simulink library "Controls_Components_lib"  (R2023b)
settings: Solver=VariableStepAuto  StartTime=0.0  StopTime=10.0  RelTol=1e-3
libraries: simulink x15, $bdroot x4, simulink_extras x3, simulink_need_slupdate x2, embmathops x1
settings Model: Creator=FIRSTMentor  LastModifiedBy=FIRSTMentor

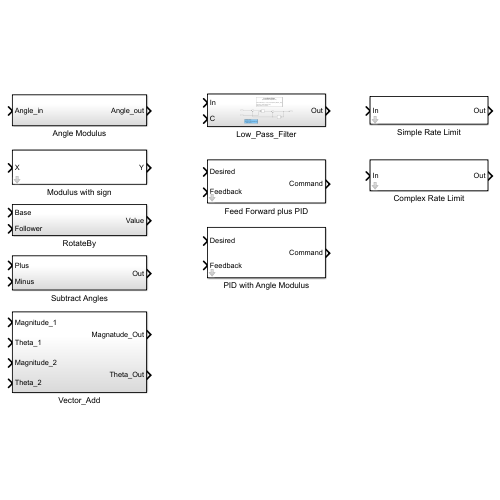
[thumbnail: Simulink's stored preview of the top-level diagram]
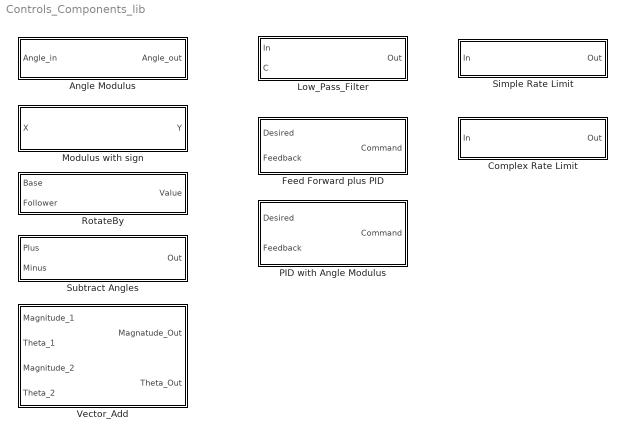
== system Controls_Components_lib ==
  Angle Modulus : Subsystem
  Complex Rate Limit : Subsystem  mask{Rate_Limit_Inc=1/0.75*0.02, Rate_Limit_Dec=-1/0.25*0.02, Approaching_Zero_Error_Threshold=0.2, Approaching_Zero_Final_Scale_Factor=0.01, Approaching_NonZero_Error_Threshold=0.2, Approaching_NonZero_Final_Scale_Factor=0.1}
  Feed Forward plus PID : Subsystem  mask{Gain_FF=1, Gain_P=1, Gain_I=1, Gain_D=1, FilterCoeff_D=0.1, Limit_I_Upper=0.1, Limit_I_Lower=-0.1, Limit_D_Upper=0.1, Limit_D_Lower=-0.1, Limit_T_Upper=1, Limit_T_Lower=-1}
      mask prompts: Gain_FF "Feed Forward Gain"; Gain_P "Proportional Gain"; Gain_I "Integral Gain"; Gain_D "Derivative Gain"; FilterCoeff_D "Derivative Filter Coefficient"; Limit_I_Upper "Integral Upper Limit"; Limit_I_Lower "Integral Lower Limit"; Limit_D_Upper "Derivative Upper Limit"; Limit_D_Lower "Derivative Lower Limit"; Limit_T_Upper "Total Command Upper Limit"; Limit_T_Lower "Total Command Lower Limit"
  Low_Pass_Filter : Subsystem
  Modulus with sign : Subsystem  mask{Number=1}
      mask prompts: Number "Enter modulus number"
  PID with Angle Modulus : Subsystem  mask{Gain_P=1, Gain_I=1, Gain_D=1, FilterCoeff_D=0.1, Limit_I_Upper=0.1, Limit_I_Lower=-0.1, Limit_D_Upper=0.1, Limit_D_Lower=-0.1, Limit_T_Upper=1, Limit_T_Lower=-1}
      mask prompts: Gain_P "Proportional Gain"; Gain_I "Integral Gain"; Gain_D "Derivative Gain"; FilterCoeff_D "Derivative Filter Coefficient"; Limit_I_Upper "Integral Upper Limit"; Limit_I_Lower "Integral Lower Limit"; Limit_D_Upper "Derivative Upper Limit"; Limit_D_Lower "Derivative Lower Limit"; Limit_T_Upper "Total Command Upper Limit"; Limit_T_Lower "Total Command Lower Limit"
  RotateBy : Subsystem
  Simple Rate Limit : Subsystem  mask{Rate_Limit_Inc=1/0.75*0.02, Rate_Limit_Dec=-1/0.25*0.02}
  Subtract Angles : Subsystem
  Vector_Add : Subsystem

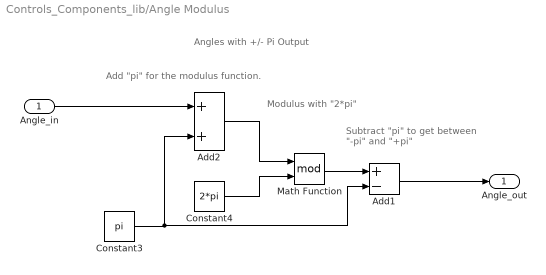
== system Controls_Components_lib/Angle Modulus ==
  note: Angles with +/- Pi Output
  note: Subtract "pi" to get
      | between "-pi" and "+pi"
  note: Modulus with "2*pi"
  note: Add "pi" for the modulus function.
  Angle_in : Inport
  Add1 : Sum  Inputs=+-
  Add2 : Sum
  Constant3 : Constant  Value=pi
  Constant4 : Constant  Value=2*pi
  Math Function : Math  Operator=mod
  Angle_out : Outport
  wires:
  Add1/1 -> Angle_out/1
  Math Function/1 -> Add1/1
  Constant4/1 -> Math Function/2
  Add2/1 -> Math Function/1
  Constant3/1 -> Add2/2, Add1/2
  Angle_in/1 -> Add2/1

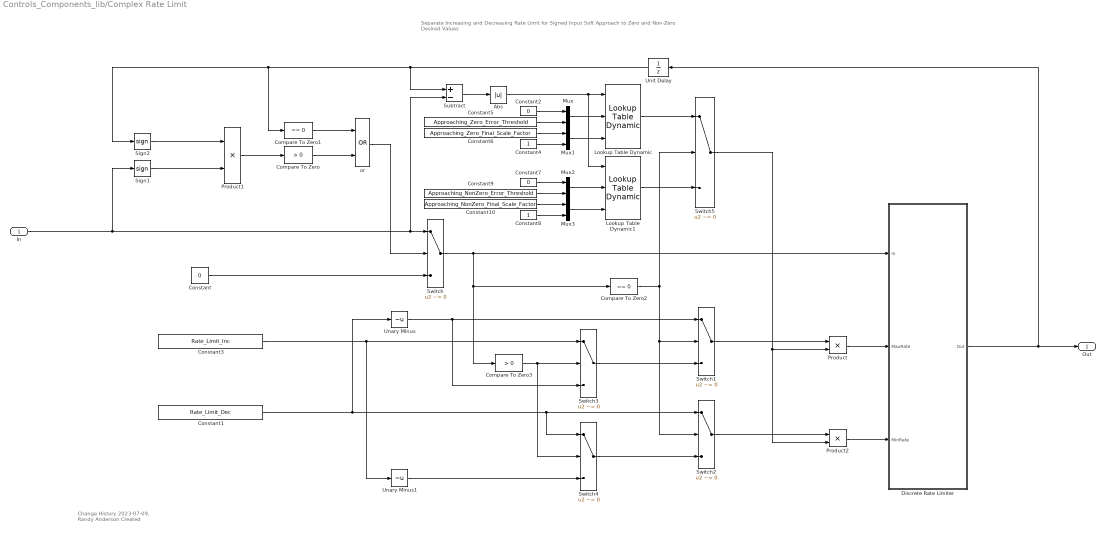
== system Controls_Components_lib/Complex Rate Limit ==
  note: Separate Increasing and Decreasing Rate Limit for Signed Input
      | Soft Approach to Zero and Non-Zero Desired Values
  note: Change History
      | 2023-07-09, Randy Anderson
      |     Created
  In : Inport
  Abs : Abs  SaturateOnIntegerOverflow=off
  Compare To Zero : simulink/Logic and Bit Operations/Compare To Zero  relop=>  OutDataTypeStr=boolean
      settings: AttributesFormatString=%<OutDataTypeStr>
  Compare To Zero1 : simulink/Logic and Bit Operations/Compare To Zero  relop===  OutDataTypeStr=boolean
      settings: AttributesFormatString=%<OutDataTypeStr>
  Compare To Zero2 : simulink/Logic and Bit Operations/Compare To Zero  relop===  OutDataTypeStr=boolean
      settings: AttributesFormatString=%<OutDataTypeStr>
  Compare To Zero3 : simulink/Logic and Bit Operations/Compare To Zero  relop=>  OutDataTypeStr=boolean
      settings: AttributesFormatString=%<OutDataTypeStr>
  Constant : Constant  Value=0  OutDataTypeStr=Inherit: Inherit via back propagation
      settings: AttributesFormatString=%<OutDataTypeStr>
  Constant1 : Constant  Value=Rate_Limit_Dec
      settings: AttributesFormatString=%<OutDataTypeStr>
  Constant10 : Constant  Value=Approaching_NonZero_Final_Scale_Factor
  Constant2 : Constant  Value=0
  Constant3 : Constant  Value=Rate_Limit_Inc
      settings: AttributesFormatString=%<OutDataTypeStr>
  Constant4 : Constant
  Constant5 : Constant  Value=Approaching_Zero_Error_Threshold
  Constant6 : Constant  Value=Approaching_Zero_Final_Scale_Factor
  Constant7 : Constant  Value=0
  Constant8 : Constant
  Constant9 : Constant  Value=Approaching_NonZero_Error_Threshold
  Discrete Rate Limiter : Subsystem
  Lookup Table Dynamic : simulink/Lookup Tables/Lookup Table Dynamic  LookUpMeth=Interpolation-Use End Values  OutDataType=fixdt('double')  OutScaling=[]  OutputDataTypeScalingMode=Specify via dialog  OutDataTypeStr=double  DoSatur=off
  Lookup Table Dynamic1 : simulink/Lookup Tables/Lookup Table Dynamic  LookUpMeth=Interpolation-Use End Values  OutDataType=fixdt('double')  OutScaling=[]  OutputDataTypeScalingMode=Specify via dialog  OutDataTypeStr=double  DoSatur=off
  Mux{,1..3} (4 alike) : Mux  Inputs=2
  Product : Product
  Product1 : Product  OutDataTypeStr=int8  RndMeth=Simplest
      settings: AttributesFormatString=Input Same DT: %<InputSameDT>\n%<OutDataTypeStr>\nSaturate: %<SaturateOnIntegerOverflow>
  Product2 : Product
  Sign1 : Signum
  Sign2 : Signum
  Subtract : Sum  Inputs=+-
  Switch{,1..4} (5 alike) : Switch  Criteria=u2 ~= 0  SaturateOnIntegerOverflow=off
      settings: AttributesFormatString=|
      | %<Criteria>
      | Input Same DT: %<InputSameDT>
      | %<OutDataTypeStr>
  Switch5 : Switch  Criteria=u2 ~= 0  SaturateOnIntegerOverflow=off  InputSameDT=off
  Unary Minus : UnaryMinus
  Unary Minus1 : UnaryMinus
  Unit Delay : UnitDelay  SampleTime=-1  HasFrameUpgradeWarning=on
      settings: AttributesFormatString=IC: %<InitialCondition>
  or : Logic  Operator=OR  OutDataTypeStr=boolean
      settings: AttributesFormatString=|
      | Input Same DT: %<AllPortsSameDT>
      | %<OutDataTypeStr>
  Out : Outport
  wires:
  Unary Minus1/1 -> Switch4/3
  Constant3/1 -> Switch3/1, Unary Minus1/1
  Unary Minus/1 -> Switch1/1, Switch3/3
  Constant1/1 -> Switch2/1, Switch4/1, Unary Minus/1
  Compare To Zero3/1 -> Switch3/2, Switch4/2
  Switch4/1 -> Switch2/3
  Switch3/1 -> Switch1/3
  Compare To Zero2/1 -> Switch2/2, Switch1/2, Switch5/2
  Compare To Zero1/1 -> or/1
  or/1 -> Switch/2
  Compare To Zero/1 -> or/2
  Discrete Rate Limiter/1(Out) -> Out/1, Unit Delay/1
  Sign1/1 -> Product1/2
  Sign2/1 -> Product1/1
  Unit Delay/1 -> Subtract/1, Compare To Zero1/1, Sign2/1
  Product1/1 -> Compare To Zero/1
  Switch/1 -> Compare To Zero2/1, Compare To Zero3/1, Discrete Rate Limiter/1(In)
  In/1 -> Sign1/1, Subtract/2, Switch/1
  Constant/1 -> Switch/3
  Switch1/1 -> Product/1
  Product/1 -> Discrete Rate Limiter/2(MaxRate)
  Product2/1 -> Discrete Rate Limiter/3(MinRate)
  Switch2/1 -> Product2/1
  Subtract/1 -> Abs/1
  Abs/1 -> Lookup Table Dynamic1/1, Lookup Table Dynamic/1
  Switch5/1 -> Product/2, Product2/2
  Lookup Table Dynamic/1 -> Switch5/1
  Mux/1 -> Lookup Table Dynamic/2
  Mux1/1 -> Lookup Table Dynamic/3
  Constant2/1 -> Mux/1
  Constant4/1 -> Mux1/2
  Constant5/1 -> Mux/2
  Constant6/1 -> Mux1/1
  Constant10/1 -> Mux3/1
  Constant9/1 -> Mux2/2
  Constant8/1 -> Mux3/2
  Constant7/1 -> Mux2/1
  Mux3/1 -> Lookup Table Dynamic1/3
  Mux2/1 -> Lookup Table Dynamic1/2
  Lookup Table Dynamic1/1 -> Switch5/3

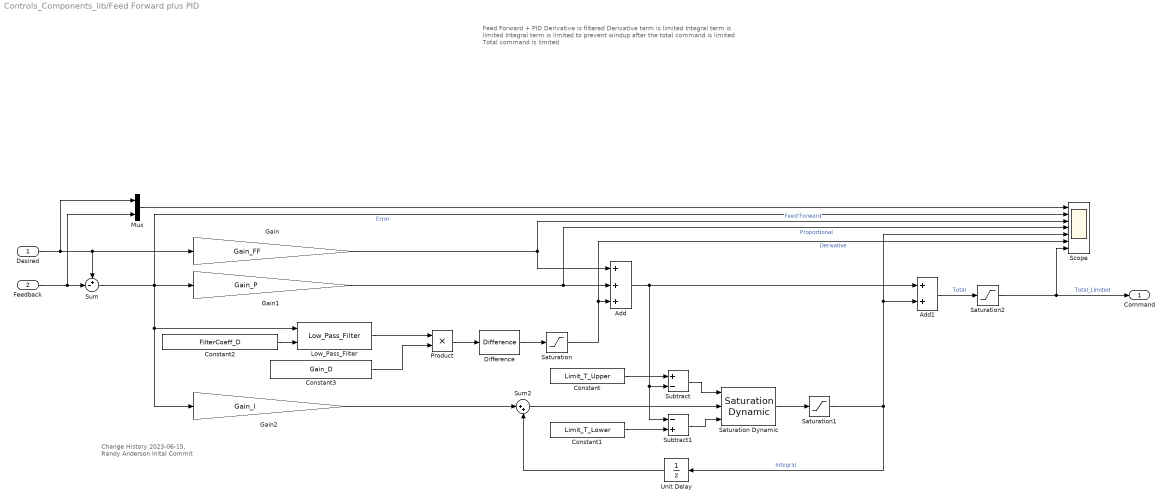
== system Controls_Components_lib/Feed Forward plus PID ==
  note: Feed Forward + PID
      |
      | Derivative is filtered
      | Derivative term is limited
      |
      | Integral term is limited
      |
      | Integral term is limited to prevent windup after the total command is limited
      |
      | Total command is limited
  note: Change History
      | 2023-06-15, Randy Anderson
      | Inital Commit
  Desired : Inport
  Feedback : Inport  Port=2
  Add : Sum  Inputs=3
  Add1 : Sum  Inputs=2
  Constant : Constant  Value=Limit_T_Upper
  Constant1 : Constant  Value=Limit_T_Lower
  Constant2 : Constant  Value=FilterCoeff_D
  Constant3 : Constant  Value=Gain_D
  Difference : simulink/Discrete/Difference  ICPrevInput=0.0  OutMin=[]  OutMax=[]  OutDataType=fixdt(1, 16)  OutScaling=2^-10  DoSatur=off
  Gain : Gain  Gain=Gain_FF
  Gain1 : Gain  Gain=Gain_P
  Gain2 : Gain  Gain=Gain_I
  Low_Pass_Filter : $bdroot/Low_Pass_Filter  SystemSampleTime=-1  VariantActivationTime=update diagram  AllowFlexibleInterface=on  Latency=0  AutoFrameSizeCalculation=off
  Mux : Mux  Inputs=2
  Product : Product
  Saturation : Saturate  UpperLimit=Limit_D_Upper  LowerLimit=Limit_D_Lower
  Saturation Dynamic : simulink/Discontinuities/Saturation Dynamic  OutMin=[]  OutMax=[]  OutDataTypeStr=Inherit: Same as second input  OutDataType=fixdt(1, 16)  OutScaling=2^-10  DoSatur=off
  Saturation1 : Saturate  UpperLimit=Limit_I_Upper  LowerLimit=Limit_I_Lower
  Saturation2 : Saturate  UpperLimit=Limit_T_Upper  LowerLimit=Limit_T_Lower
  Scope : Scope  NumInputPorts=7
  Subtract : Sum  Inputs=+-
  Subtract1 : Sum  Inputs=-+
  Sum : Sum  Inputs=+-|
  Sum2 : Sum  Inputs=|++
  Unit Delay : UnitDelay  SampleTime=-1  HasFrameUpgradeWarning=on
  Command : Outport
  wires:
  Sum/1 -> Gain2/1, Low_Pass_Filter/1, Gain1/1, Scope/2  "Error"
  Gain/1 -> Add/1, Scope/3  "Feed Forward"
  Add/1 -> Add1/1, Subtract1/1, Subtract/2
  Subtract1/1 -> Saturation Dynamic/3
  Gain1/1 -> Add/2, Scope/4  "Proportional"
  Gain2/1 -> Sum2/1
  Saturation Dynamic/1 -> Saturation1/1
  Subtract/1 -> Saturation Dynamic/1
  Unit Delay/1 -> Sum2/2
  Constant/1 -> Subtract/1
  Constant1/1 -> Subtract1/2
  Add1/1 -> Saturation2/1  "Total"
  Desired/1 -> Mux/1, Sum/1, Gain/1
  Difference/1 -> Saturation/1
  Saturation/1 -> Scope/6, Add/3  "Derivative"
  Product/1 -> Difference/1
  Low_Pass_Filter/1 -> Product/1
  Constant2/1 -> Low_Pass_Filter/2
  Constant3/1 -> Product/2
  Sum2/1 -> Saturation Dynamic/2
  Feedback/1 -> Mux/2, Sum/2
  Saturation2/1 -> Scope/7, Command/1  "Total_Limited"
  Saturation1/1 -> Unit Delay/1, Scope/5, Add1/2  "Integral"
  Mux/1 -> Scope/1

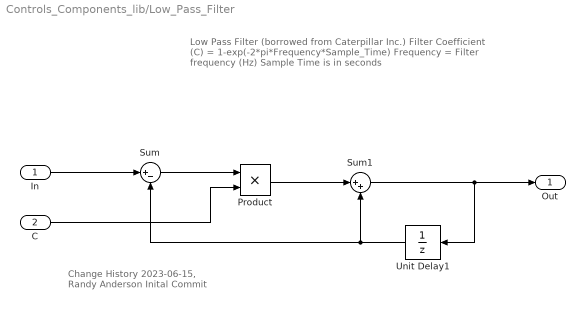
== system Controls_Components_lib/Low_Pass_Filter ==
  note: Low Pass Filter
      | (borrowed from Caterpillar Inc.)
      |
      | Filter Coefficient (C) = 1-exp(-2*pi*Frequency*Sample_Time)
      |
      | Frequency = Filter frequency (Hz)
      | Sample Time is in seconds
  note: Change History
      | 2023-06-15, Randy Anderson
      | Inital Commit
  In : Inport
  C : Inport  Port=2
  Product : Product
  Sum : Sum  Inputs=|+-
  Sum1 : Sum  Inputs=|++
  Unit Delay1 : UnitDelay  SampleTime=-1  HasFrameUpgradeWarning=on
  Out : Outport
  wires:
  In/1 -> Sum/1
  Sum1/1 -> Out/1, Unit Delay1/1
  Product/1 -> Sum1/1
  Unit Delay1/1 -> Sum/2, Sum1/2
  Sum/1 -> Product/1
  C/1 -> Product/2

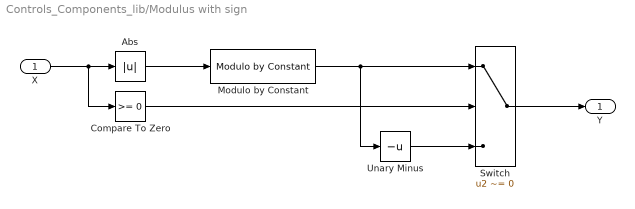
== system Controls_Components_lib/Modulus with sign ==
  X : Inport
  Abs : Abs  SaturateOnIntegerOverflow=off
  Compare To Zero : simulink/Logic and Bit Operations/Compare To Zero  relop=>=  OutDataTypeStr=boolean
  Modulo by Constant : embmathops/Modulo by Constant  Denominator=Number  SimulateUsing=Code generation
      settings: LibrarySourceBlock=embeddedMathLib/Modulo by Constant
  Switch : Switch  Criteria=u2 ~= 0  SaturateOnIntegerOverflow=off  InputSameDT=off
  Unary Minus : UnaryMinus
  Y : Outport
  wires:
  X/1 -> Compare To Zero/1, Abs/1
  Abs/1 -> Modulo by Constant/1
  Switch/1 -> Y/1
  Modulo by Constant/1 -> Unary Minus/1, Switch/1
  Unary Minus/1 -> Switch/3
  Compare To Zero/1 -> Switch/2

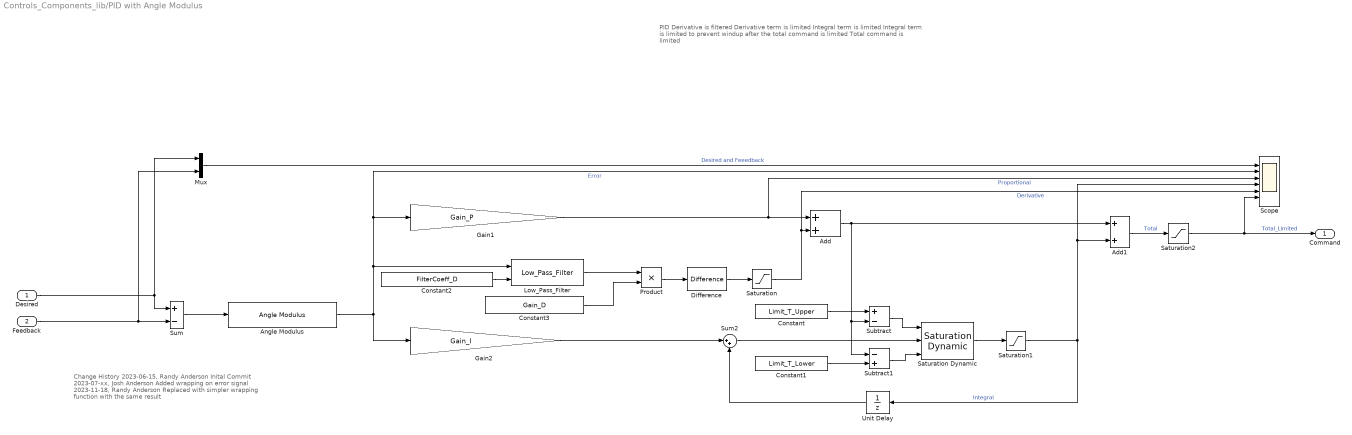
== system Controls_Components_lib/PID with Angle Modulus ==
  note: PID
      |
      | Derivative is filtered
      | Derivative term is limited
      |
      | Integral term is limited
      |
      | Integral term is limited to prevent windup after the total command is limited
      |
      | Total command is limited
  note: Change History
      | 2023-06-15, Randy Anderson
      | Inital Commit
      | 2023-07-xx, Josh Anderson
      | Added wrapping on error signal
      | 2023-11-18, Randy Anderson
      | Replaced with simpler wrapping function with the same result
  Desired : Inport
  Feedback : Inport  Port=2
  Add : Sum  Inputs=2
  Add1 : Sum  Inputs=2
  Angle Modulus : $bdroot/Angle Modulus  SystemSampleTime=-1  VariantActivationTime=update diagram  AllowFlexibleInterface=on  Latency=0  AutoFrameSizeCalculation=off
  Constant : Constant  Value=Limit_T_Upper
  Constant1 : Constant  Value=Limit_T_Lower
  Constant2 : Constant  Value=FilterCoeff_D
  Constant3 : Constant  Value=Gain_D
  Difference : simulink/Discrete/Difference  ICPrevInput=0.0  OutMin=[]  OutMax=[]  OutDataType=fixdt(1, 16)  OutScaling=2^-10  DoSatur=off
  Gain1 : Gain  Gain=Gain_P
  Gain2 : Gain  Gain=Gain_I
  Low_Pass_Filter : $bdroot/Low_Pass_Filter  SystemSampleTime=-1  VariantActivationTime=update diagram  AllowFlexibleInterface=on  Latency=0  AutoFrameSizeCalculation=off
  Mux : Mux  Inputs=2
  Product : Product
  Saturation : Saturate  UpperLimit=Limit_D_Upper  LowerLimit=Limit_D_Lower
  Saturation Dynamic : simulink/Discontinuities/Saturation Dynamic  OutMin=[]  OutMax=[]  OutDataTypeStr=Inherit: Same as second input  OutDataType=fixdt(1, 16)  OutScaling=2^-10  DoSatur=off
  Saturation1 : Saturate  UpperLimit=Limit_I_Upper  LowerLimit=Limit_I_Lower
  Saturation2 : Saturate  UpperLimit=Limit_T_Upper  LowerLimit=Limit_T_Lower
  Scope : Scope  NumInputPorts=6
  Subtract : Sum  Inputs=+-
  Subtract1 : Sum  Inputs=-+
  Sum : Sum  Inputs=+-
  Sum2 : Sum  Inputs=|++
  Unit Delay : UnitDelay  SampleTime=-1  HasFrameUpgradeWarning=on
  Command : Outport
  wires:
  Angle Modulus/1 -> Gain1/1, Scope/2, Low_Pass_Filter/1, Gain2/1  "Error"
  Add/1 -> Subtract1/1, Subtract/2, Add1/1
  Subtract1/1 -> Saturation Dynamic/3
  Gain1/1 -> Scope/3, Add/1  "Proportional"
  Gain2/1 -> Sum2/1
  Saturation Dynamic/1 -> Saturation1/1
  Subtract/1 -> Saturation Dynamic/1
  Unit Delay/1 -> Sum2/2
  Constant/1 -> Subtract/1
  Constant1/1 -> Subtract1/2
  Add1/1 -> Saturation2/1  "Total"
  Desired/1 -> Mux/1, Sum/1
  Difference/1 -> Saturation/1
  Saturation/1 -> Scope/5, Add/2  "Derivative"
  Product/1 -> Difference/1
  Low_Pass_Filter/1 -> Product/1
  Constant2/1 -> Low_Pass_Filter/2
  Constant3/1 -> Product/2
  Sum2/1 -> Saturation Dynamic/2
  Feedback/1 -> Mux/2, Sum/2
  Saturation2/1 -> Scope/6, Command/1  "Total_Limited"
  Saturation1/1 -> Unit Delay/1, Scope/4, Add1/2  "Integral"
  Mux/1 -> Scope/1  "Desired and Feeedback"
  Sum/1 -> Angle Modulus/1

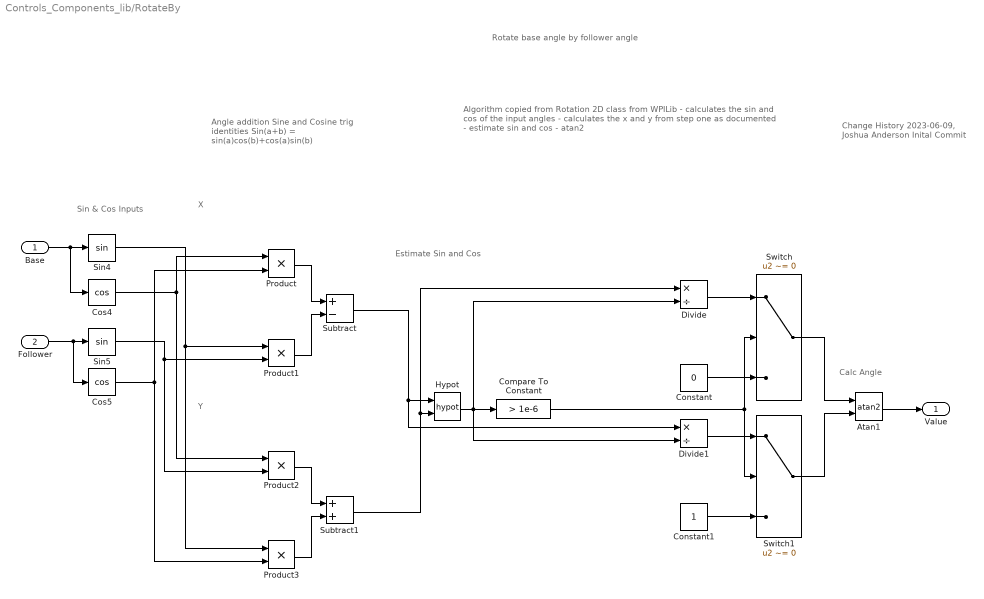
== system Controls_Components_lib/RotateBy ==
  note: Sin & Cos
      | Inputs
  note: Calc Angle
  note: Estimate Sin and Cos
  note: Angle addition Sine and Cosine trig identities
      |
      | Sin(a+b) = sin(a)cos(b)+cos(a)sin(b)
  note: Y
  note: X
  note: Algorithm copied from Rotation 2D class from WPILib
      | - calculates the sin and cos of the input angles
      | - calculates the x and y from step one as documented
      | - estimate sin and cos
      | - atan2
  note: Change History
      | 2023-06-09, Joshua Anderson
      | Inital Commit
  note: Rotate base angle by follower angle
  Base : Inport  OutDataTypeStr=double  Unit=rad
  Follower : Inport  Port=2  OutDataTypeStr=double  Unit=rad
  Atan1 : Trigonometry  Operator=atan2
  Compare To Constant : simulink/Logic and Bit Operations/Compare To Constant  relop=>  const=1e-6  OutDataTypeStr=boolean
  Constant : Constant  Value=0
  Constant1 : Constant
  Cos4 : Trigonometry  Operator=cos
  Cos5 : Trigonometry  Operator=cos
  Divide : Product  Inputs=*/
  Divide1 : Product  Inputs=*/
  Hypot : Math  Operator=hypot
  Product{,1..3} (4 alike) : Product
  Sin4 : Trigonometry
  Sin5 : Trigonometry
  Subtract : Sum  Inputs=+-
  Subtract1 : Sum
  Switch : Switch  Criteria=u2 ~= 0  SaturateOnIntegerOverflow=off  InputSameDT=off
  Switch1 : Switch  Criteria=u2 ~= 0  SaturateOnIntegerOverflow=off  InputSameDT=off
  Value : Outport  OutDataTypeStr=double  Unit=rad
  wires:
  Product/1 -> Subtract/1
  Product1/1 -> Subtract/2
  Sin5/1 -> Product2/2, Product1/2
  Cos5/1 -> Product/2, Product3/2
  Product2/1 -> Subtract1/1
  Cos4/1 -> Product/1, Product2/1
  Product3/1 -> Subtract1/2
  Sin4/1 -> Product3/1, Product1/1
  Atan1/1 -> Value/1
  Subtract/1 -> Divide1/1, Hypot/1
  Subtract1/1 -> Divide/1, Hypot/2
  Hypot/1 -> Compare To Constant/1, Divide/2, Divide1/2
  Switch/1 -> Atan1/1
  Switch1/1 -> Atan1/2
  Constant/1 -> Switch/3
  Constant1/1 -> Switch1/3
  Compare To Constant/1 -> Switch1/2, Switch/2
  Divide/1 -> Switch/1
  Divide1/1 -> Switch1/1
  Base/1 -> Cos4/1, Sin4/1
  Follower/1 -> Cos5/1, Sin5/1

== system Controls_Components_lib/Simple Rate Limit ==
  note: Change History
      | 2023-07-10, Randy Anderson
      |     Created
  note: Simple Rate Limit
  In : Inport
  Constant1 : Constant  Value=Rate_Limit_Dec
      settings: AttributesFormatString=%<OutDataTypeStr>
  Constant3 : Constant  Value=Rate_Limit_Inc
      settings: AttributesFormatString=%<OutDataTypeStr>
  Discrete Rate Limiter : Subsystem
  Out : Outport
  wires:
  Discrete Rate Limiter/1(Out) -> Out/1
  In/1 -> Discrete Rate Limiter/1(In)
  Constant3/1 -> Discrete Rate Limiter/2(MaxRate)
  Constant1/1 -> Discrete Rate Limiter/3(MinRate)

== system Controls_Components_lib/Subtract Angles ==
  note: Subtract angles by flipping the sign of argument 2 and using the rotate by function to effectivly add the inverse.
  note: Change History
      | 2023-06-09, Joshua Anderson
      | Inital Commit
  note: Subtract angles
  Plus : Inport
  Minus : Inport  Port=2
  RotateBy : $bdroot/RotateBy  SystemSampleTime=-1  VariantActivationTime=update diagram  AllowFlexibleInterface=on  Latency=0  AutoFrameSizeCalculation=off
  Unary Minus : UnaryMinus
  Out : Outport
  wires:
  Plus/1 -> RotateBy/1
  RotateBy/1 -> Out/1
  Minus/1 -> Unary Minus/1
  Unary Minus/1 -> RotateBy/2

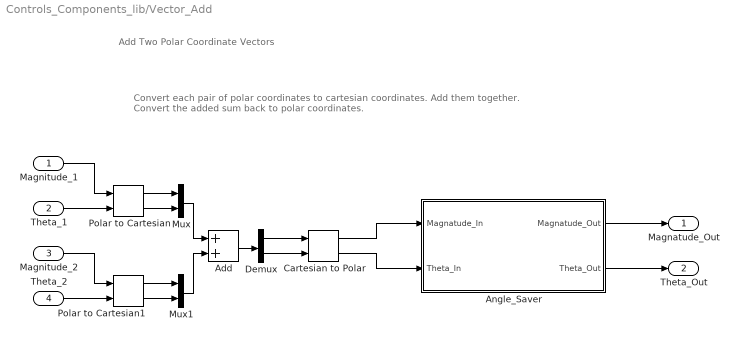
== system Controls_Components_lib/Vector_Add ==
  note: Convert each pair of polar coordinates to cartesian coordinates.
      | Add them together.
      | Convert the added sum back to polar coordinates.
  note: Add Two Polar Coordinate Vectors
  Magnitude_1 : Inport
  Theta_1 : Inport  Port=2
  Magnitude_2 : Inport  Port=3
  Theta_2 : Inport  Port=4
  Add : Sum
  Angle_Saver : Subsystem
  Cartesian to Polar : simulink_extras/Transformations/Cartesian to Polar
  Demux : Demux  Outputs=2
  Mux : Mux  Inputs=2
  Mux1 : Mux  Inputs=2
  Polar to Cartesian : simulink_extras/Transformations/Polar to Cartesian
  Polar to Cartesian1 : simulink_extras/Transformations/Polar to Cartesian
  Magnatude_Out : Outport
  Theta_Out : Outport  Port=2
  wires:
  Cartesian to Polar/1 -> Angle_Saver/1(Magnatude_In)
  Theta_2/1 -> Polar to Cartesian1/2
  Theta_1/1 -> Polar to Cartesian/2
  Magnitude_2/1 -> Polar to Cartesian1/1
  Magnitude_1/1 -> Polar to Cartesian/1
  Polar to Cartesian/1 -> Mux/1
  Polar to Cartesian/2 -> Mux/2
  Polar to Cartesian1/2 -> Mux1/2
  Polar to Cartesian1/1 -> Mux1/1
  Mux/1 -> Add/1
  Mux1/1 -> Add/2
  Add/1 -> Demux/1
  Demux/1 -> Cartesian to Polar/1
  Demux/2 -> Cartesian to Polar/2
  Cartesian to Polar/2 -> Angle_Saver/2(Theta_In)
  Angle_Saver/2(Theta_Out) -> Theta_Out/1
  Angle_Saver/1(Magnatude_Out) -> Magnatude_Out/1

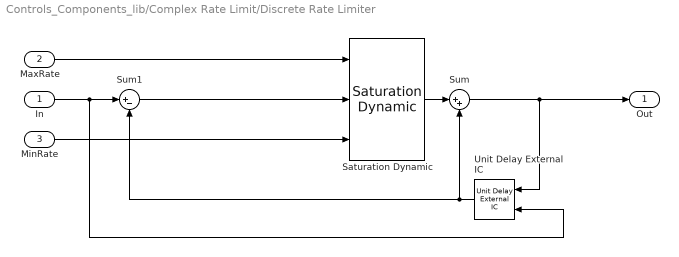
== system Controls_Components_lib/Complex Rate Limit/Discrete Rate Limiter ==
  In : Inport
  MaxRate : Inport  Port=2
  MinRate : Inport  Port=3
  Saturation Dynamic : simulink/Discontinuities/Saturation Dynamic  OutMin=[]  OutMax=[]  OutDataTypeStr=Inherit: Same as second input  OutDataType=fixdt(1, 16)  OutScaling=2^-10  DoSatur=off
  Sum : Sum  Inputs=|++  OutDataTypeStr=Inherit: Inherit via back propagation
  Sum1 : Sum  Inputs=|+-  OutDataTypeStr=Inherit: Inherit via back propagation  SaturateOnIntegerOverflow=on
  Unit Delay External IC : simulink_need_slupdate/Unit Delay External IC  tsamp=-1
  Out : Outport
  wires:
  Sum/1 -> Out/1, Unit Delay External IC/1
  MinRate/1 -> Saturation Dynamic/3
  MaxRate/1 -> Saturation Dynamic/1
  Saturation Dynamic/1 -> Sum/1
  Sum1/1 -> Saturation Dynamic/2
  Unit Delay External IC/1 -> Sum1/2, Sum/2
  In/1 -> Unit Delay External IC/2, Sum1/1

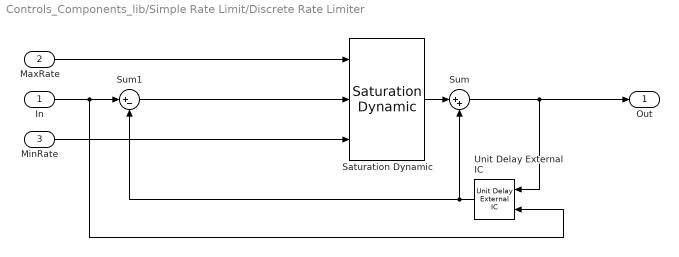
== system Controls_Components_lib/Simple Rate Limit/Discrete Rate Limiter ==
  In : Inport
  MaxRate : Inport  Port=2
  MinRate : Inport  Port=3
  Saturation Dynamic : simulink/Discontinuities/Saturation Dynamic  OutMin=[]  OutMax=[]  OutDataTypeStr=Inherit: Same as second input  OutDataType=fixdt(1, 16)  OutScaling=2^-10  DoSatur=off
  Sum : Sum  Inputs=|++  OutDataTypeStr=Inherit: Inherit via back propagation
  Sum1 : Sum  Inputs=|+-  OutDataTypeStr=Inherit: Inherit via back propagation  SaturateOnIntegerOverflow=on
  Unit Delay External IC : simulink_need_slupdate/Unit Delay External IC  tsamp=-1
  Out : Outport
  wires:
  In/1 -> Sum1/1, Unit Delay External IC/2
  Unit Delay External IC/1 -> Sum/2, Sum1/2
  Sum1/1 -> Saturation Dynamic/2
  Saturation Dynamic/1 -> Sum/1
  MaxRate/1 -> Saturation Dynamic/1
  MinRate/1 -> Saturation Dynamic/3
  Sum/1 -> Unit Delay External IC/1, Out/1

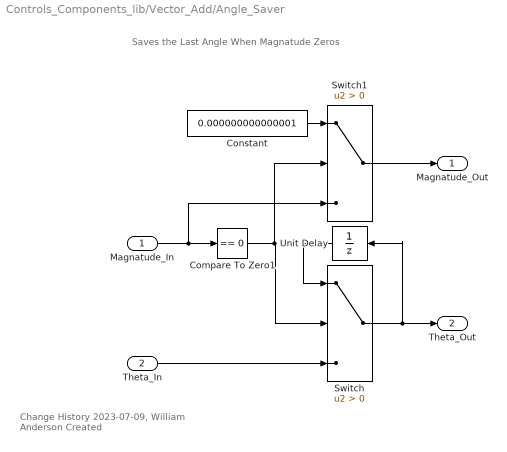
== system Controls_Components_lib/Vector_Add/Angle_Saver ==
  note: Change History
      | 2023-07-09, William Anderson
      | Created
  note: Saves the Last Angle When Magnatude Zeros
  Magnatude_In : Inport
  Theta_In : Inport  Port=2
  Compare To Zero1 : simulink/Logic and Bit Operations/Compare To Zero  relop===  OutDataTypeStr=boolean
  Constant : Constant  Value=0.000000000000001
  Switch : Switch  Criteria=u2 > Threshold  SaturateOnIntegerOverflow=off  InputSameDT=off
  Switch1 : Switch  Criteria=u2 > Threshold  SaturateOnIntegerOverflow=off  InputSameDT=off
  Unit Delay : UnitDelay  SampleTime=-1  HasFrameUpgradeWarning=on
  Magnatude_Out : Outport
  Theta_Out : Outport  Port=2
  wires:
  Magnatude_In/1 -> Switch1/3, Compare To Zero1/1
  Switch/1 -> Unit Delay/1, Theta_Out/1
  Unit Delay/1 -> Switch/1
  Compare To Zero1/1 -> Switch1/2, Switch/2
  Switch1/1 -> Magnatude_Out/1
  Theta_In/1 -> Switch/3
  Constant/1 -> Switch1/1
